simulink model "Level2Sfunc_simulink"  (R2022b)
settings: Solver=VariableStepAuto  StartTime=0.0  StopTime=10.0  RelTol=1e-3
settings Model: Creator=chris  LastModifiedBy=chris

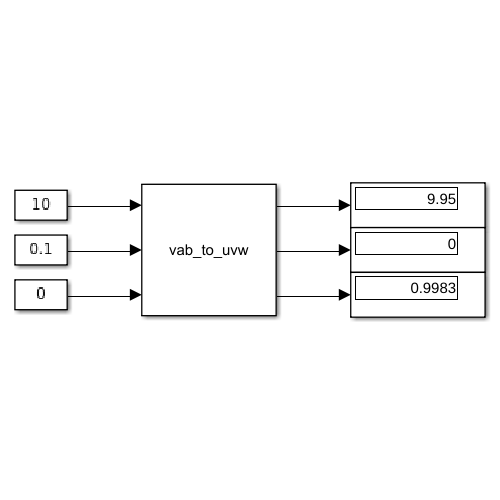
[thumbnail: Simulink's stored preview of the top-level diagram]
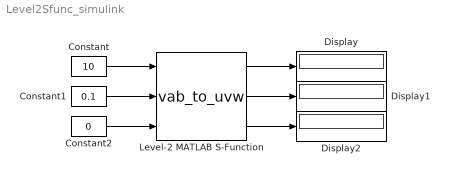
== system Level2Sfunc_simulink ==
  Constant : Constant  Value=10
  Constant1 : Constant  Value=0.1
  Constant2 : Constant  Value=0
  Display : Display
  Display1 : Display
  Display2 : Display
  Level-2 MATLAB S-Function : M-S-Function  FunctionName=vab_to_uvw
  wires:
  Constant/1 -> Level-2 MATLAB S-Function/1
  Constant1/1 -> Level-2 MATLAB S-Function/2
  Constant2/1 -> Level-2 MATLAB S-Function/3
  Level-2 MATLAB S-Function/1 -> Display/1
  Level-2 MATLAB S-Function/2 -> Display1/1
  Level-2 MATLAB S-Function/3 -> Display2/1
